simulink model "verify_Radiator_AIV_mdl"  (R2016b)
settings: Solver=ode45  StartTime=0  StopTime=8*3600  MaxStep=600  RelTol=1e-3  EnableMultiTasking=on
InitFcn:
  | load('DE_TRY2010_13_averageYear')
libraries: carnot x5, simulink x1
settings Model: Creator=drhf  LastModifiedBy=User
settings DataIOCC: SaveFormat=Array  SignalLoggingSaveFormat=ModelDataLogs
settings OptimizationCC: ExpressionDepthLimit=2147483647  LifeSpan=inf
settings DebuggingCC: UnderspecifiedInitializationDetection=Classic  MergeDetectMultiDrivingBlocksExec=none  SolverPrmCheckMsg=warning  FcnCallInpInsideContextMsg=warning  StateNameClashWarn=warning  SFUnexpectedBacktrackingDiag=warning  SFNoUnconditionalDefaultTransitionDiag=warning  SFExecutionAtInitializationDiag=none
settings HardwareCC: ProdBitPerPointer=32  ProdBitPerSizeT=32  ProdBitPerPtrDiffT=32  ProdLargestAtomicFloat=None  ProdIntDivRoundTo=Undefined  ProdEndianess=Unspecified  ProdWordSize=32  ProdHWDeviceType=32-bit Generic
settings ModelReferenceCC: PropagateSignalLabelsOutOfModel=off
settings GRTTargetCC: TargetLangStandard=C89/C90 (ANSI)  GeneratePreprocessorConditionals=Disable all  CombineOutputUpdateFcns=off  GRTInterface=on
settings ConfigComp: CovMetricSettings=dw  CovHtmlReporting=on  CovSaveCumulativeToWorkspaceVar=on  CovSaveSingleToWorkspaceVar=on  CovExternalEMLEnable=off

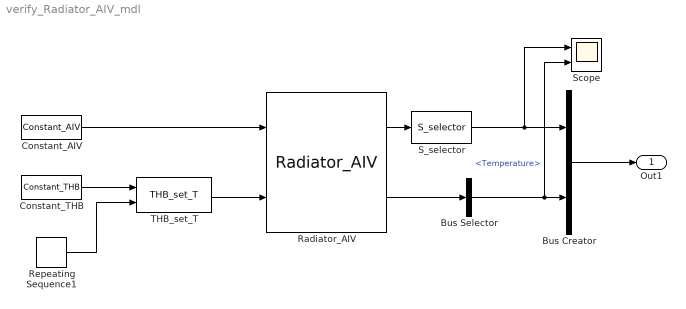
== system verify_Radiator_AIV_mdl ==
  Bus Creator : BusCreator  Inputs=2
  Bus Selector : BusSelector  OutputSignals=Temperature
  Constant_AIV : carnot/Source/Ventilation/Constant_AIV  Tsens=20  Tcon=20  Trad=20  mw=0.012  mco=0.01  rhoair=1.2  cpair=1004  pair=100000  nair=0.5
  Constant_THB : carnot/Source/Simple/Constant_THB  t=40  mdot=1000/4182/10  p=1e5  mID=No Pressure Drop  fluid=Water (Constant 20°C)  mix=0  mix2=0  mix3=0  dia=0.02  hgt=0
  Radiator_AIV : carnot/Source/Heat_Exchanger/Radiator_AIV  pnom=500  dtnom=40  expo=1.3  mcap=5*4182  ra=0.47  tini=20  lin=10  qua=10
  Repeating Sequence1 : simulink/Sources/Repeating Sequence  rep_seq_t=[0 2 2.1 4 4.1 6 6.1 8]*3600  rep_seq_y=[45 45 55 55 65 65 75 75]
  S_selector : carnot/Outputs/S_selector  e1=off  e2=off  e3=off  e4=off  e5=on  e6=off  e7=off  e8=off  e9=off  e10=off  e11=off  e12=off  e13=off
  Scope : Scope  NumInputPorts=2
  THB_set_T : carnot/Source/Simple/THB_set_T
  Out1 : Outport
  wires:
  Bus Creator/1 -> Out1/1
  Radiator_AIV/2 -> Bus Selector/1
  Constant_THB/1 -> THB_set_T/1
  Repeating Sequence1/1 -> THB_set_T/2
  THB_set_T/1 -> Radiator_AIV/2
  Radiator_AIV/1 -> S_selector/1
  Bus Selector/1 -> Scope/2, Bus Creator/2  "<Temperature>"
  Constant_AIV/1 -> Radiator_AIV/1
  S_selector/1 -> Scope/1, Bus Creator/1
